simulink model "questao2_pat_estimador"  (R2020a)
settings: Solver=VariableStepAuto  StartTime=0.0  StopTime=50  RelTol=1e-3
values from neighbouring files (symbols this model uses):
  A = [1 2 0;-1 -1 -1;0 2 -1]    [lqr_estudos.m]    (also in questao2_pat.m = [1 2 0; -1 -1 -1; 0 2 -1])
  Alc = A - L * C    [questao1_pat.m]    (also in questao2_pat.m)
  B = [0;0;2]    [lqr_estudos.m]    (also in questao2_pat.m)
  C = [0 1 0;0 0 1]    [lqr_estudos.m]    (also in questao2_pat.m = [0 1 0; 0 0 1])
  K = place(A,B,poles)    [estudos_versao_laurinda.m]    (also in lqr_estudos.m = lqr(A,B,Q,R); questao1_pat.m = Ka(1:3); questao1_well.m = Ka(1:3); questao2_pat.m = lqr(A, B, Q, R))
  L = L'    [questao1_pat.m]    (also in questao2_pat.m)
  N = -1/(C*inv(Acl-B*K)*B)    [questao2_pat.m]
settings Model: Creator=wwagner  LastModifiedBy=patricia

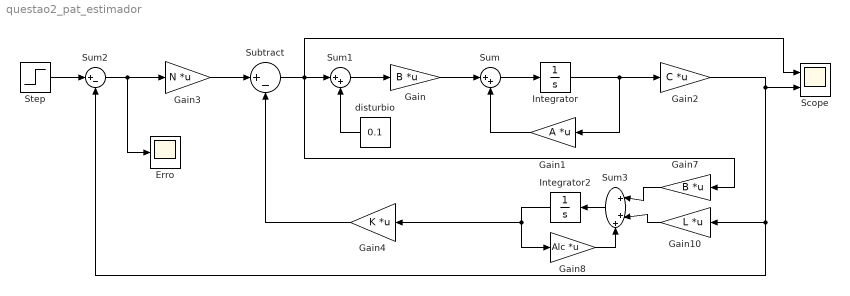
== system questao2_pat_estimador ==
  Erro : Scope
  Gain : Gain  Gain=B  Multiplication=Matrix(K*u)
  Gain1 : Gain  Gain=A  Multiplication=Matrix(K*u)
  Gain10 : Gain  Gain=L  Multiplication=Matrix(K*u)
  Gain2 : Gain  Gain=C  Multiplication=Matrix(K*u)
  Gain3 : Gain  Gain=N  Multiplication=Matrix(K*u)
  Gain4 : Gain  Gain=K  Multiplication=Matrix(K*u)
  Gain7 : Gain  Gain=B  Multiplication=Matrix(K*u)
  Gain8 : Gain  Gain=Alc  Multiplication=Matrix(K*u)
  Integrator : Integrator
  Integrator2 : Integrator
  Scope : Scope  NumInputPorts=2
  Step : Step  SampleTime=0
  Subtract : Sum  Inputs=|+-
  Sum : Sum  Inputs=|++
  Sum1 : Sum  Inputs=|++
  Sum2 : Sum  Inputs=|+-
  Sum3 : Sum  Inputs=|+++
  disturbio : Constant  Value=0.1
  wires:
  Integrator/1 -> Gain2/1, Gain1/1
  Gain/1 -> Sum/1
  Gain1/1 -> Sum/2
  Sum/1 -> Integrator/1
  Gain2/1 -> Scope/2, Gain10/1, Sum2/2
  Sum1/1 -> Gain/1
  Sum2/1 -> Gain3/1, Erro/1
  Subtract/1 -> Scope/1, Gain7/1, Sum1/1
  Gain7/1 -> Sum3/1
  Integrator2/1 -> Gain4/1, Gain8/1
  Gain10/1 -> Sum3/2
  Sum3/1 -> Integrator2/1
  Gain8/1 -> Sum3/3
  Step/1 -> Sum2/1
  disturbio/1 -> Sum1/2
  Gain3/1 -> Subtract/1
  Gain4/1 -> Subtract/2
